simulink model "testing_loop"  (R2016b)
settings: Solver=VariableStepAuto  StartTime=0.0  StopTime=10.0  RelTol=1e-3
undefined symbols (not defined in the file or in its folder): sigbuilder_block
libraries: link_test x1
settings Model: Creator=Harjot  LastModifiedBy=Harjot

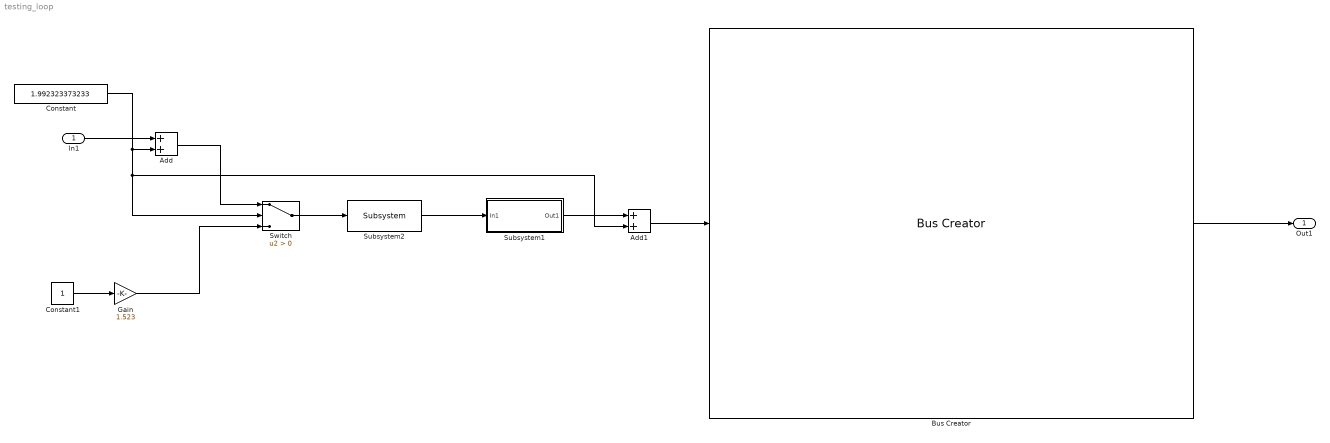
== system testing_loop ==
  In1 : Inport
  Add : Sum
  Add1 : Sum
  Bus Creator : BusCreator  Inputs=1
  Constant : Constant  Value=1.992323373233
  Constant1 : Constant
  Gain : Gain  Gain=1.523
  Subsystem1 : Subsystem
  Subsystem2 : link_test/Subsystem
  Switch : Switch  Criteria=u2 > Threshold
  Out1 : Outport
  wires:
  In1/1 -> Add/1
  Add/1 -> Switch/1
  Constant/1 -> Add1/2, Switch/2, Add/2
  Constant1/1 -> Gain/1
  Gain/1 -> Switch/3
  Switch/1 -> Subsystem2/1
  Subsystem2/1 -> Subsystem1/1(In1)
  Subsystem1/1(Out1) -> Add1/1
  Add1/1 -> Bus Creator/1
  Bus Creator/1 -> Out1/1

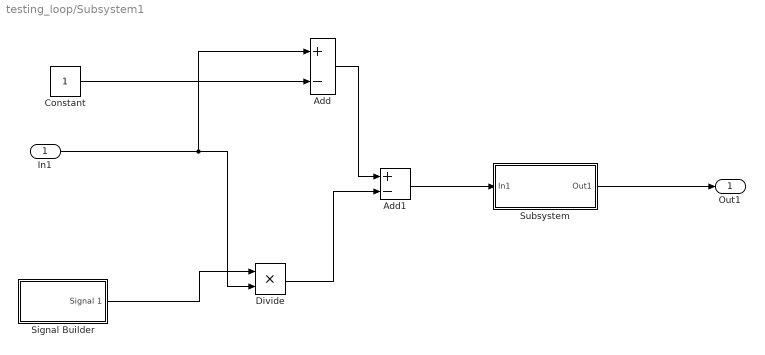
== system testing_loop/Subsystem1 ==
  In1 : Inport
  Add : Sum  Inputs=+-
  Add1 : Sum  Inputs=+-
  Constant : Constant
  Divide : Product  Inputs=**
  Signal Builder : Subsystem  Tag=STV Subsys  LoadFcn=sigbuilder_block('load');  StartFcn=sigbuilder_block('start');  StopFcn=sigbuilder_block('stop');  ClipboardFcn=sigbuilder_block('clipboard');  mask(Sigbuilder block){tuvar=[0:10]}
      mask help: Simulink:masks:SigbuilderBlock_MD
      mask init:
      | if ~strcmp(get_param(bdroot(gcbh),'SimulationStatus'),'stopped') tuvar = sigbuilder_block('maskInit'); end
      settings: CopyFcn=sigbuilder_block('copy');  DeleteFcn=sigbuilder_block('delete');  ModelCloseFcn=sigbuilder_block('modelClose');  PreSaveFcn=sigbuilder_block('preSave');  PauseFcn=sigbuilder_block('pause');  ContinueFcn=sigbuilder_block('continue');  NameChangeFcn=sigbuilder_block('namechange');  OpenFcn=sigbuilder_block('open',[349.8 80.4 550.8 400.2 ]);  CloseFcn=sigbuilder_block('close');
      mask Display: plot(0, 0, 100, 100,[2, 2, 32, 32, 2], [68, 8, 8, 68, 68],[32, 2], [38, 38], [32, 19, 2],[53, 60, 44], [32, 17, 17, 2],[16, 16, 31, 31]);txt = getActiveGroup(gcbh);text(2, 100, txt,'verticalAlignment', 'top');
  Subsystem : Subsystem
  Out1 : Outport
  wires:
  Signal Builder/1(Signal 1) -> Divide/1
  In1/1 -> Add/1, Divide/2
  Constant/1 -> Add/2
  Add/1 -> Add1/1
  Divide/1 -> Add1/2
  Add1/1 -> Subsystem/1(In1)
  Subsystem/1(Out1) -> Out1/1

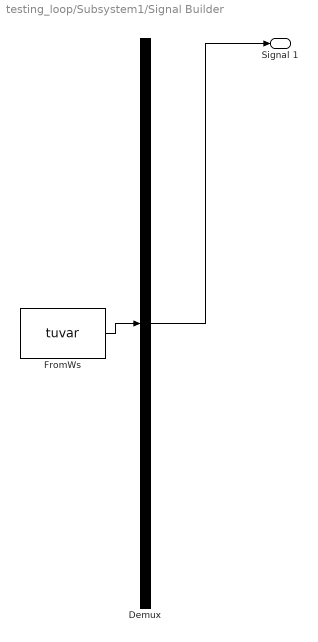
== system testing_loop/Subsystem1/Signal Builder ==
  Demux : Demux  Tag=STV Demux  Outputs=1
  FromWs : FromWorkspace  Tag=STV FromWs  VariableName=tuvar  SampleTime=0
      SigBuilderData=|
      | common.afterFinalStr = 'Extrapolate'
      | common.sampleTime = 0
      | dataSet.timeRange = [0 10]
      | dataSet.name = 'Group 1'
      | sbobj.Groups.Name = 'Group 1'
      | sbobj.Groups.Signals.Name = 'Signal 1'
      | sbobj.Groups.Signals.XData = [0 4 4 6 6 10]
      | sbobj.Groups.Signals.YData = [0 0 1 1 0 0]
  Signal 1 : Outport  Tag=STV Outport
  wires:
  Demux/1 -> Signal 1/1
  FromWs/1 -> Demux/1

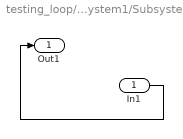
== system testing_loop/Subsystem1/Subsystem ==
  In1 : Inport
  Out1 : Outport
  wires:
  In1/1 -> Out1/1
